simulink model "Joystick_Demo"  (R2024b)
settings: Solver=VariableStepAuto  StartTime=0.0  StopTime=t_final  RelTol=1e-3
libraries: vrlib x1, aerolibanimutils x1
settings Model: Creator=jaspergeldenbott  LastModifiedBy=jaspergeldenbott

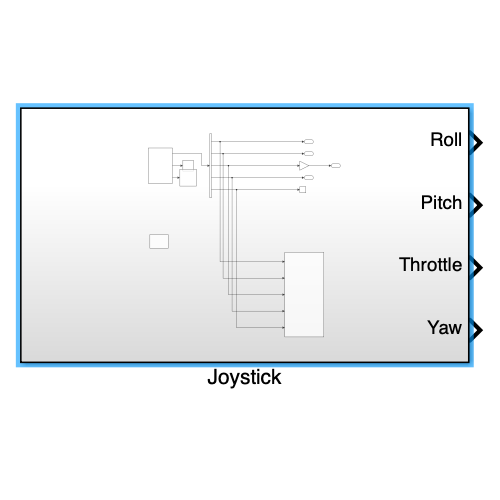
[thumbnail: Simulink's stored preview of the top-level diagram]
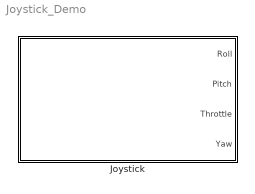
== system Joystick_Demo ==
  Joystick : Subsystem

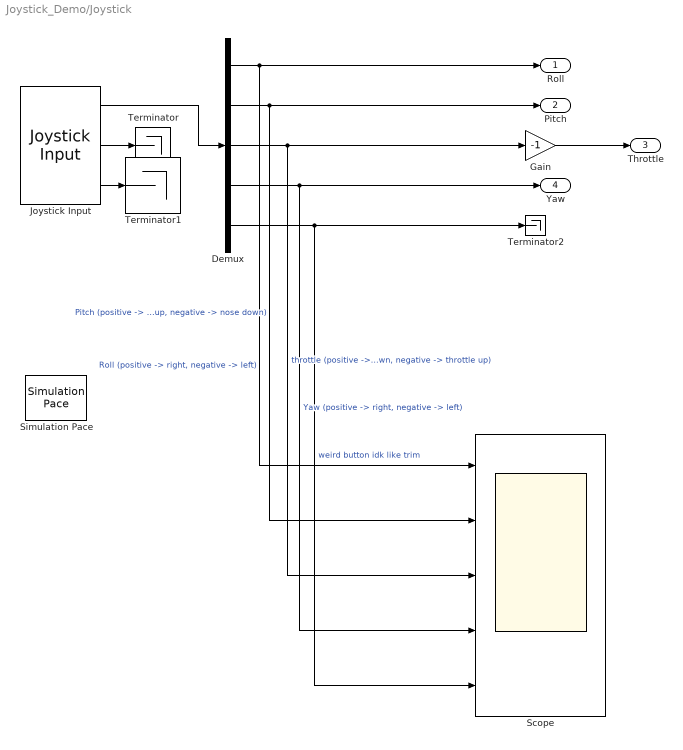
== system Joystick_Demo/Joystick ==
  Demux : Demux  Outputs=5
  Gain : Gain  Gain=-1
  Joystick Input : vrlib/Joystick Input  joyid=0  adjustports=on  forcefeed=off
  Scope : Scope  NumInputPorts=5
  Simulation Pace : aerolibanimutils/Simulation Pace  SimulationPace=1  SleepMode=Auto  OutputPaceError=off  SampleTime=1/50
  Terminator : Terminator
  Terminator1 : Terminator
  Terminator2 : Terminator
  Roll : Outport
  Pitch : Outport  Port=2
  Throttle : Outport  Port=3
  Yaw : Outport  Port=4
  wires:
  Gain/1 -> Throttle/1
  Demux/4 -> Scope/4, Yaw/1  "Yaw (positive -> right, negative -> left)"
  Demux/2 -> Scope/2, Pitch/1  "Pitch (positive -> nose up, negative -> nose down)"
  Joystick Input/3 -> Terminator1/1
  Demux/3 -> Scope/3, Gain/1  "throttle (positive -> throttle down, negative -> throttle up)"
  Joystick Input/1 -> Demux/1
  Joystick Input/2 -> Terminator/1
  Demux/1 -> Scope/1, Roll/1  "Roll (positive -> right, negative -> left)"
  Demux/5 -> Scope/5, Terminator2/1  "weird button idk like trim"
